simulink model "edrive"  (R2016b)
settings: Solver=ode1  StartTime=0.0  StopTime=1  FixedStep=ctrlConst.TsSim  MaxStep=1e-6  RelTol=1e-3  EnableMultiTasking=on
PreLoadFcn:
  | %rtwdemo_pmsmfoc_data
StartFcn:
  | %clear executionProfile
StopFcn:
  | %try
  | %  AddExecutionProfileToDataInspector();
  | %end
undefined symbols (not defined in the file or in its folder): canChannel, ctrlConst, ECM, EGM, hm11, hm13, hm5, hm7, Np, pmsm, sensors, sldrtexcb_modeswitch, SpdSetTest, theta0, TrqSetTest, Ts_10ms, Tsw
libraries: powerlib x26, canmsglib x23, simulink x14, canlib x12, powerlib_extras x9
(part 4 of 4)

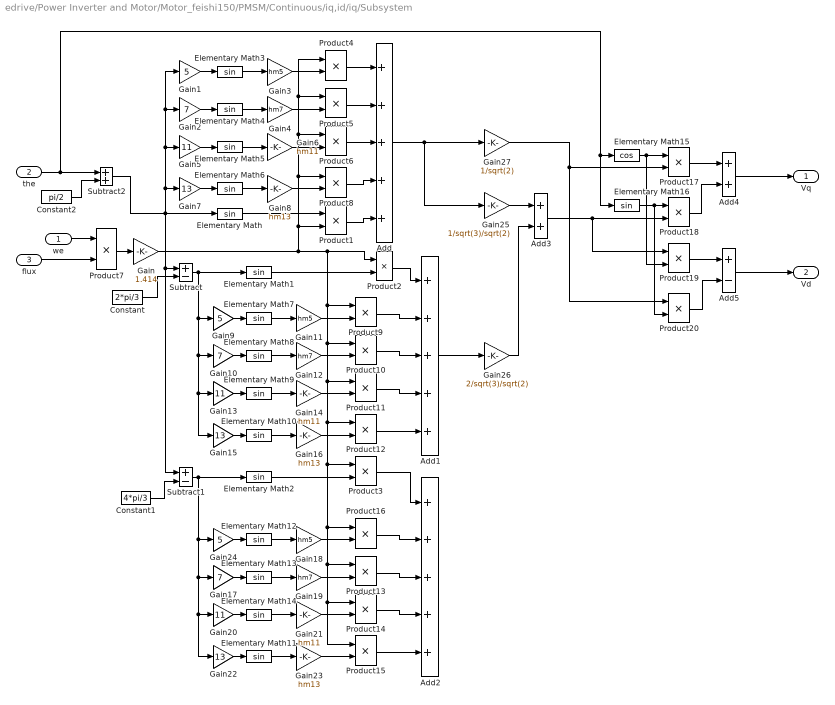
== system edrive/Power Inverter and Motor/Motor_feishi150/PMSM/Continuous/iq,id/iq/Subsystem ==
  we : Inport
  the : Inport  Port=2
  flux : Inport  Port=3
  Add : Sum  Inputs=+++++
  Add1 : Sum  Inputs=+++++
  Add2 : Sum  Inputs=+++++
  Add3 : Sum
  Add4 : Sum
  Add5 : Sum  Inputs=+-
  Constant : Constant  Value=2*pi/3
  Constant1 : Constant  Value=4*pi/3
  Constant2 : Constant  Value=pi/2
  Elementary Math{,1..14,16} (16 alike) : Trigonometry
  Elementary Math15 : Trigonometry  Operator=cos
  Gain : Gain  Gain=1.414  SaturateOnIntegerOverflow=on  OutDataTypeStr=Inherit: Same as input  ParamDataTypeStr=Inherit: Same as input
  Gain1 : Gain  Gain=5  SaturateOnIntegerOverflow=on  OutDataTypeStr=Inherit: Same as input  ParamDataTypeStr=Inherit: Same as input
  Gain10 : Gain  Gain=7  SaturateOnIntegerOverflow=on  OutDataTypeStr=Inherit: Same as input  ParamDataTypeStr=Inherit: Same as input
  Gain11 : Gain  Gain=hm5  SaturateOnIntegerOverflow=on  OutDataTypeStr=Inherit: Same as input  ParamDataTypeStr=Inherit: Same as input
  Gain12 : Gain  Gain=hm7  SaturateOnIntegerOverflow=on  OutDataTypeStr=Inherit: Same as input  ParamDataTypeStr=Inherit: Same as input
  Gain13 : Gain  Gain=11  SaturateOnIntegerOverflow=on  OutDataTypeStr=Inherit: Same as input  ParamDataTypeStr=Inherit: Same as input
  Gain14 : Gain  Gain=hm11  SaturateOnIntegerOverflow=on  OutDataTypeStr=Inherit: Same as input  ParamDataTypeStr=Inherit: Same as input
  Gain15 : Gain  Gain=13  SaturateOnIntegerOverflow=on  OutDataTypeStr=Inherit: Same as input  ParamDataTypeStr=Inherit: Same as input
  Gain16 : Gain  Gain=hm13  SaturateOnIntegerOverflow=on  OutDataTypeStr=Inherit: Same as input  ParamDataTypeStr=Inherit: Same as input
  Gain17 : Gain  Gain=7  SaturateOnIntegerOverflow=on  OutDataTypeStr=Inherit: Same as input  ParamDataTypeStr=Inherit: Same as input
  Gain18 : Gain  Gain=hm5  SaturateOnIntegerOverflow=on  OutDataTypeStr=Inherit: Same as input  ParamDataTypeStr=Inherit: Same as input
  Gain19 : Gain  Gain=hm7  SaturateOnIntegerOverflow=on  OutDataTypeStr=Inherit: Same as input  ParamDataTypeStr=Inherit: Same as input
  Gain2 : Gain  Gain=7  SaturateOnIntegerOverflow=on  OutDataTypeStr=Inherit: Same as input  ParamDataTypeStr=Inherit: Same as input
  Gain20 : Gain  Gain=11  SaturateOnIntegerOverflow=on  OutDataTypeStr=Inherit: Same as input  ParamDataTypeStr=Inherit: Same as input
  Gain21 : Gain  Gain=hm11  SaturateOnIntegerOverflow=on  OutDataTypeStr=Inherit: Same as input  ParamDataTypeStr=Inherit: Same as input
  Gain22 : Gain  Gain=13  SaturateOnIntegerOverflow=on  OutDataTypeStr=Inherit: Same as input  ParamDataTypeStr=Inherit: Same as input
  Gain23 : Gain  Gain=hm13  SaturateOnIntegerOverflow=on  OutDataTypeStr=Inherit: Same as input  ParamDataTypeStr=Inherit: Same as input
  Gain24 : Gain  Gain=5  SaturateOnIntegerOverflow=on  OutDataTypeStr=Inherit: Same as input  ParamDataTypeStr=Inherit: Same as input
  Gain25 : Gain  Gain=1/sqrt(3)/sqrt(2)  SaturateOnIntegerOverflow=on  OutDataTypeStr=Inherit: Same as input  ParamDataTypeStr=Inherit: Same as input
  Gain26 : Gain  Gain=2/sqrt(3)/sqrt(2)  SaturateOnIntegerOverflow=on  OutDataTypeStr=Inherit: Same as input  ParamDataTypeStr=Inherit: Same as input
  Gain27 : Gain  Gain=1/sqrt(2)  SaturateOnIntegerOverflow=on  OutDataTypeStr=Inherit: Same as input  ParamDataTypeStr=Inherit: Same as input
  Gain3 : Gain  Gain=hm5  SaturateOnIntegerOverflow=on  OutDataTypeStr=Inherit: Same as input  ParamDataTypeStr=Inherit: Same as input
  Gain4 : Gain  Gain=hm7  SaturateOnIntegerOverflow=on  OutDataTypeStr=Inherit: Same as input  ParamDataTypeStr=Inherit: Same as input
  Gain5 : Gain  Gain=11  SaturateOnIntegerOverflow=on  OutDataTypeStr=Inherit: Same as input  ParamDataTypeStr=Inherit: Same as input
  Gain6 : Gain  Gain=hm11  SaturateOnIntegerOverflow=on  OutDataTypeStr=Inherit: Same as input  ParamDataTypeStr=Inherit: Same as input
  Gain7 : Gain  Gain=13  SaturateOnIntegerOverflow=on  OutDataTypeStr=Inherit: Same as input  ParamDataTypeStr=Inherit: Same as input
  Gain8 : Gain  Gain=hm13  SaturateOnIntegerOverflow=on  OutDataTypeStr=Inherit: Same as input  ParamDataTypeStr=Inherit: Same as input
  Gain9 : Gain  Gain=5  SaturateOnIntegerOverflow=on  OutDataTypeStr=Inherit: Same as input  ParamDataTypeStr=Inherit: Same as input
  Product{1..20} (20 alike) : Product  Inputs=**  SaturateOnIntegerOverflow=on  InputSameDT=on  OutDataTypeStr=Inherit: Same as first input
  Subtract : Sum  Inputs=+-
  Subtract1 : Sum  Inputs=+-
  Subtract2 : Sum
  Vq : Outport  InitialOutput=0
  Vd : Outport  Port=2  InitialOutput=0
  wires:
  flux/1 -> Product7/2
  Product7/1 -> Gain/1
  we/1 -> Product7/1
  Elementary Math/1 -> Product1/1
  Product1/1 -> Add/5
  Subtract/1 -> Gain9/1, Gain15/1, Gain13/1, Gain10/1, Elementary Math1/1
  Constant/1 -> Subtract/2
  Constant1/1 -> Subtract1/2
  Elementary Math1/1 -> Product2/2
  Elementary Math2/1 -> Product3/2
  Gain1/1 -> Elementary Math3/1
  Gain2/1 -> Elementary Math4/1
  Elementary Math3/1 -> Gain3/1
  Elementary Math4/1 -> Gain4/1
  Gain5/1 -> Elementary Math5/1
  Elementary Math5/1 -> Gain6/1
  Subtract2/1 -> Gain1/1, Gain2/1, Gain5/1, Gain7/1, Subtract1/1, Subtract/1, Elementary Math/1
  Gain7/1 -> Elementary Math6/1
  Elementary Math6/1 -> Gain8/1
  Gain3/1 -> Product4/2
  Gain4/1 -> Product5/2
  Gain6/1 -> Product6/2
  Gain8/1 -> Product8/2
  Product4/1 -> Add/1
  Product5/1 -> Add/2
  Product6/1 -> Add/3
  Product8/1 -> Add/4
  Add/1 -> Gain27/1, Gain25/1
  Gain9/1 -> Elementary Math7/1
  Gain10/1 -> Elementary Math8/1
  Elementary Math7/1 -> Gain11/1
  Elementary Math8/1 -> Gain12/1
  Gain13/1 -> Elementary Math9/1
  Elementary Math9/1 -> Gain14/1
  Gain15/1 -> Elementary Math10/1
  Elementary Math10/1 -> Gain16/1
  Gain11/1 -> Product9/2
  Gain12/1 -> Product10/2
  Gain14/1 -> Product11/2
  Gain16/1 -> Product12/2
  Gain/1 -> Product1/2, Product8/1, Product6/1, Product5/1, Product4/1, Product12/1, Product3/1, Product16/1, Product13/1, Product14/1, Product15/1, Product11/1, Product10/1, Product9/1, Product2/1
  Product9/1 -> Add1/2
  Product10/1 -> Add1/3
  Product11/1 -> Add1/4
  Product12/1 -> Add1/5
  Product2/1 -> Add1/1
  Add1/1 -> Gain26/1
  Subtract1/1 -> Gain24/1, Gain22/1, Gain20/1, Gain17/1, Elementary Math2/1
  Gain24/1 -> Elementary Math12/1
  Gain17/1 -> Elementary Math13/1
  Elementary Math12/1 -> Gain18/1
  Elementary Math13/1 -> Gain19/1
  Gain20/1 -> Elementary Math14/1
  Elementary Math14/1 -> Gain21/1
  Gain18/1 -> Product16/2
  Gain19/1 -> Product13/2
  Gain21/1 -> Product14/2
  Product16/1 -> Add2/2
  Product13/1 -> Add2/3
  Product14/1 -> Add2/4
  Product15/1 -> Add2/5
  Gain23/1 -> Product15/2
  Product3/1 -> Add2/1
  Elementary Math11/1 -> Gain23/1
  Gain22/1 -> Elementary Math11/1
  Gain25/1 -> Add3/1
  Gain26/1 -> Add3/2
  Add3/1 -> Product19/1, Product18/2
  Elementary Math15/1 -> Product19/2, Product17/1
  Elementary Math16/1 -> Product20/2, Product18/1
  Product17/1 -> Add4/1
  Product18/1 -> Add4/2
  Product19/1 -> Add5/1
  Product20/1 -> Add5/2
  Add5/1 -> Vd/1
  the/1 -> Elementary Math15/1, Elementary Math16/1, Subtract2/1
  Constant2/1 -> Subtract2/2
  Add4/1 -> Vq/1
  Gain27/1 -> Product20/1, Product17/2

== matlab function edrive/Motor Control Board/Hardware platform/Motor Control Board ==
  data: MR_ON input; KL30 output; KL30_1 output; bCtlSmps input; bLoEnFen input; bHiEnFen input; VDD15 output; VDD15Fb output; RelsHiDfw input; RelsLoDfw input; RDY_H output; RDY_L output; modHiIgbtDrv input; modLoIgbtDrv input; LvMoCSOP output; HvMoCSOP output; stIgbtDrvCnfgOk output; modIgbtDrvL1 output; modIgbtDrvL2 output; modIgbtDrvL3 output; modIgbtDrvH1 output; modIgbtDrvH2 output; modIgbtDrvH3 output
function [KL30,KL30_1,VDD15,VDD15Fb,RDY_H,RDY_L,LvMoCSOP,HvMoCSOP,stIgbtDrvCnfgOk,...
    modIgbtDrvL1,modIgbtDrvL2,modIgbtDrvL3,modIgbtDrvH1,modIgbtDrvH2,modIgbtDrvH3]...
    = fcn(MR_ON,bCtlSmps,bLoEnFen,bHiEnFen,RelsHiDfw,RelsLoDfw,modHiIgbtDrv,modLoIgbtDrv)
%
persistent modTmpIgbtDrvL1;
persistent modTmpIgbtDrvL2;
persistent modTmpIgbtDrvL3;
persistent modTmpIgbtDrvH1;
persistent modTmpIgbtDrvH2;
persistent modTmpIgbtDrvH3;
persistent HvMoCSOPTmp;
persistent stIgbtDrvCnfgOkTmp;

if isempty(modTmpIgbtDrvL1)
    modTmpIgbtDrvL1 = EiceSilOPM.OPM0;
    modTmpIgbtDrvL2 = EiceSilOPM.OPM0;
    modTmpIgbtDrvL3 = EiceSilOPM.OPM0;
    modTmpIgbtDrvH1 = EiceSilOPM.OPM0;
    modTmpIgbtDrvH2 = EiceSilOPM.OPM0;
    modTmpIgbtDrvH3 = EiceSilOPM.OPM0;
    HvMoCSOPTmp = false;
    stIgbtDrvCnfgOkTmp = false;
end

if MR_ON
    KL30 = 12;
    KL30_1 = 12;  
    
    if bCtlSmps   %12 to 16V boost/buck on
        VDD15 = 16;
        
        if RelsLoDfw
            RDY_L = true;
            if modLoIgbtDrv==EiceSilSM.EsTarMod5
                modTmpIgbtDrvL1 = EiceSilOPM.OPM5;
                modTmpIgbtDrvL2 = EiceSilOPM.OPM5;
                modTmpIgbtDrvL3 = EiceSilOPM.OPM5;
            elseif modLoIgbtDrv==EiceSilSM.EsTarMod3
                modTmpIgbtDrvL1 = EiceSilOPM.OPM3;
                modTmpIgbtDrvL2 = EiceSilOPM.OPM3;
                modTmpIgbtDrvL3 = EiceSilOPM.OPM3;
            elseif modLoIgbtDrv==EiceSilSM.EsReadSts
                if bLoEnFen
                    if modTmpIgbtDrvL1==EiceSilOPM.OPM5
                        modTmpIgbtDrvL1 = EiceSilOPM.OPM6;
                        modTmpIgbtDrvL2 = EiceSilOPM.OPM6;
                        modTmpIgbtDrvL3 = EiceSilOPM.OPM6;
                    elseif modTmpIgbtDrvL1==EiceSilOPM.OPM3
                        modTmpIgbtDrvL1 = EiceSilOPM.OPM4;
                        modTmpIgbtDrvL2 = EiceSilOPM.OPM4;
                        modTmpIgbtDrvL3 = EiceSilOPM.OPM4;
                    end
                end
            end   
        else
            RDY_L = false;
        end
        
        if RelsHiDfw
            RDY_H = true;
            if modHiIgbtDrv==EiceSilSM.EsTarMod5
                modTmpIgbtDrvH1 = EiceSilOPM.OPM5;
                modTmpIgbtDrvH2 = EiceSilOPM.OPM5;
                modTmpIgbtDrvH3 = EiceSilOPM.OPM5;
            elseif modHiIgbtDrv==EiceSilSM.EsTarMod3
                modTmpIgbtDrvH1 = EiceSilOPM.OPM3;
                modTmpIgbtDrvH2 = EiceSilOPM.OPM3;
                modTmpIgbtDrvH3 = EiceSilOPM.OPM3;
            elseif modHiIgbtDrv==EiceSilSM.EsReadSts
                if bHiEnFen
                    if modTmpIgbtDrvH1==EiceSilOPM.OPM5
                        modTmpIgbtDrvH1 = EiceSilOPM.OPM6;
                        modTmpIgbtDrvH2 = EiceSilOPM.OPM6;
                        modTmpIgbtDrvH3 = EiceSilOPM.OPM6;
                    elseif modTmpIgbtDrvH1==EiceSilOPM.OPM3
                        modTmpIgbtDrvH1 = EiceSilOPM.OPM4;
                        modTmpIgbtDrvH2 = EiceSilOPM.OPM4;
                        modTmpIgbtDrvH3 = EiceSilOPM.OPM4;
                    end
                end
            end
        else
            RDY_H = false;
        end
    else
        VDD15 = 0;
        RDY_L = false;
        RDY_H = false;
    end
    
    if RDY_H&&RDY_L  %Lv mocsop
        LvMoCSOP = true;
    else
        LvMoCSOP = false;
    end
    
    if (modTmpIgbtDrvH1==EiceSilOPM.OPM6)&&(modTmpIgbtDrvL1==EiceSilOPM.OPM6)
        HvMoCSOPTmp = true;
        stIgbtDrvCnfgOkTmp = true;
    end
else
    KL30 = 0;
    KL30_1 = 0;  
    VDD15 = 0;
    RDY_H = false;
    RDY_L = false;
    LvMoCSOP = false;
    HvMoCSOPTmp = false;
    stIgbtDrvCnfgOkTmp = false;
end

modIgbtDrvL1 = modTmpIgbtDrvL1;
modIgbtDrvL2 = modTmpIgbtDrvL2;
modIgbtDrvL3 = modTmpIgbtDrvL3;
modIgbtDrvH1 = modTmpIgbtDrvH1;
modIgbtDrvH2 = modTmpIgbtDrvH2;
modIgbtDrvH3 = modTmpIgbtDrvH3;
HvMoCSOP = HvMoCSOPTmp;
stIgbtDrvCnfgOk = stIgbtDrvCnfgOkTmp;
VDD15Fb = 0;

== matlab function edrive/Power Inverter and Motor/Inverter/Measure/PswCal ==
  data: ia input; ib input; ic input; iba input; ibb input; ibc input; Psw output; Udc input; Idc_add output
function [Psw,Idc_add] = PswCal(ia,ib,ic,iba,ibb,ibc,Udc)

if iba>2
    Psw_a = 0.059*abs(ia);   %mJ,Eon+Erec=41.3mJ/700A
elseif iba>(-2)
    Psw_a = 0;
else
    Psw_a = 0.0908*abs(ia);  %mJ,Eoff=63.6mJ/700A
end

if ibb>2
    Psw_b = 0.059*abs(ib);   %mJ,Eon+Erec=41.3mJ/700A
elseif ibb>(-2)
    Psw_b = 0;
else
    Psw_b = 0.0908*abs(ib);  %mJ,Eoff=63.6mJ/700A
end

if ibc>2
    Psw_c = 0.059*abs(ic);   %mJ,Eon+Erec=41.3mJ/700A
elseif ibc>(-2)
    Psw_c = 0;
else
    Psw_c = 0.0908*abs(ic);  %mJ,Eoff=63.6mJ/700A
end

Psw = (Psw_a + Psw_b + Psw_c)*1000; %to Power
Idc_add = Psw/Udc;

== matlab function edrive/System Analysis/Measure/Eff Cal ==
  data: m_power input; e_power input; eff output
function eff  = Eff_cal(m_power,e_power)

if m_power>0
    eff = m_power/e_power;
else
    eff = abs(e_power)/abs(m_power);
end

== matlab function edrive/Motor Control Board/GTM/SVPWMtoDuty/Generate pulse pattern/GTM_Hi ==
  data: Cnt input; Port output; tiOn input; tiOff input
function Port = fcn(Cnt,tiOn,tiOff)
%
persistent Port_Last; 
if isempty(Port_Last)
    Port_Last = 0;
end

if tiOn<tiOff
    if Cnt<tiOn
        Port = Port_Last;
    elseif Cnt<tiOff
        Port = 1;
    else
        Port = 0;
    end
else
    if Cnt<tiOff
        Port = Port_Last;
    elseif Cnt<tiOn
        Port = 0;
    else
        Port = 1;
    end
end

Port_Last = Port;

== matlab function edrive/Motor Control Board/GTM/SVPWMtoDuty/Generate pulse pattern1/GTM_Hi ==
  data: Cnt input; Port output; tiOn input; tiOff input
function Port = fcn(Cnt,tiOn,tiOff)
%
persistent Port_Last; 
if isempty(Port_Last)
    Port_Last = 0;
end

if tiOn<tiOff
    if Cnt<tiOn
        Port = Port_Last;
    elseif Cnt<tiOff
        Port = 1;
    else
        Port = 0;
    end
else
    if Cnt<tiOff
        Port = Port_Last;
    elseif Cnt<tiOn
        Port = 0;
    else
        Port = 1;
    end
end

Port_Last = Port;

== matlab function edrive/Motor Control Board/GTM/SVPWMtoDuty/Generate pulse pattern2/GTM_Hi ==
  data: Cnt input; Port output; tiOn input; tiOff input
function Port = fcn(Cnt,tiOn,tiOff)
%
persistent Port_Last; 
if isempty(Port_Last)
    Port_Last = 0;
end

if tiOn<tiOff
    if Cnt<tiOn
        Port = Port_Last;
    elseif Cnt<tiOff
        Port = 1;
    else
        Port = 0;
    end
else
    if Cnt<tiOff
        Port = Port_Last;
    elseif Cnt<tiOn
        Port = 0;
    else
        Port = 1;
    end
end

Port_Last = Port;

== matlab function edrive/Motor Control Board/GTM/SVPWMtoDuty/Generate pulse pattern3/GTM_Lo ==
  data: Cnt input; tiOff input; Port output; tiOn input
function Port = fcn(Cnt,tiOff,tiOn)
%
persistent Port_Last; 
if isempty(Port_Last)
    Port_Last = 1;
end

if tiOff<tiOn
    if Cnt<tiOff
        Port = Port_Last;
    elseif Cnt<tiOn
        Port = 0;
    else
        Port = 1;
    end
else
    if Cnt<tiOn
        Port = Port_Last;
    elseif Cnt<tiOff
        Port = 1;
    else
        Port = 0;
    end
end

Port_Last = Port;

== matlab function edrive/Motor Control Board/GTM/SVPWMtoDuty/Generate pulse pattern4/GTM_Lo ==
  data: Cnt input; tiOff input; Port output; tiOn input
function Port = fcn(Cnt,tiOff,tiOn)
%
persistent Port_Last; 
if isempty(Port_Last)
    Port_Last = 1;
end

if tiOff<tiOn
    if Cnt<tiOff
        Port = Port_Last;
    elseif Cnt<tiOn
        Port = 0;
    else
        Port = 1;
    end
else
    if Cnt<tiOn
        Port = Port_Last;
    elseif Cnt<tiOff
        Port = 1;
    else
        Port = 0;
    end
end

Port_Last = Port;

== matlab function edrive/Motor Control Board/GTM/SVPWMtoDuty/Generate pulse pattern5/GTM_Lo ==
  data: Cnt input; tiOff input; Port output; tiOn input
function Port = fcn(Cnt,tiOff,tiOn)
%
persistent Port_Last; 
if isempty(Port_Last)
    Port_Last = 1;
end

if tiOff<tiOn
    if Cnt<tiOff
        Port = Port_Last;
    elseif Cnt<tiOn
        Port = 0;
    else
        Port = 1;
    end
else
    if Cnt<tiOn
        Port = Port_Last;
    elseif Cnt<tiOff
        Port = 1;
    else
        Port = 0;
    end
end

Port_Last = Port;

== matlab function edrive/System Analysis/System test/test ==
  data: torqueSet input; torque_act input; out output
function out  = m_10ms(torqueSet,torque_act)

if abs(torqueSet-torque_act)<5
    out = uint8(1);
else
    out = uint8(0);
end
